simulink model "NPC_IM_YT"  (R2017b)
settings: Solver=ode45  StartTime=0.0  StopTime=5  MaxStep=1e-6  RelTol=1e-3
libraries: powerlib x35
settings Model: Creator=sibly  LastModifiedBy=alfonso
settings CodeAppCC: StateflowObjectComments=on
settings SimscapeCC: SimscapeNormalizeSystem=off

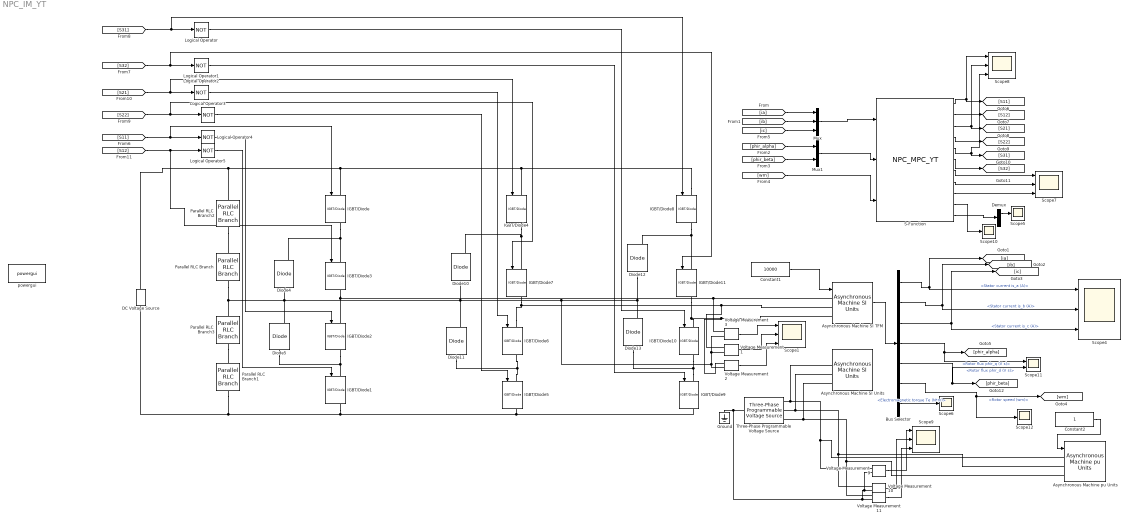
== system NPC_IM_YT ==
  Asynchronous Machine SI TFM : powerlib/Machines/Asynchronous Machine SI Units  RotorType=Squirrel-cage  PresetModel=No  MechanicalLoad=Torque Tm  ShowDetailedParameters=on  ReferenceFrame=Stationary  Units=SI  MeasurementBus=off  NominalParameters=[2035e3 3300 50]  Stator=[0.05761 0.002544]  Rotor=[0.04889 0.001881]  Cage1=[0.4155 0.002066]  Cage2=[0.4168 0.0003495]  Lm=0.04001  Mechanical=[42.14 0 5]  PolePairs=2  InitialConditions=[0 0 0 0 0 0 0 0]  SimulateSaturation=off  Saturation=[14.03593122, 27.81365428, 53.79336849, 72.68890987, 97.98006896, 148.6815601, 215.7428561, 302.9841135, 428.7778367 ; 230, 322, 414, 460, 506, 552, 598, 644, 690]  LoadFlowParameters=1492000  TsPowergui=0  TsBlock=-1  IterativeModel=Trapezoidal non iterative  IterativeDiscreteModel=Trapezoidal non iterative  Pmec=1.587e6
  Asynchronous Machine SI Units : powerlib/Machines/Asynchronous Machine SI Units  RotorType=Squirrel-cage  PresetModel=No  MechanicalLoad=Torque Tm  ShowDetailedParameters=on  ReferenceFrame=Stationary  Units=SI  MeasurementBus=off  NominalParameters=[7000 460 60]  Stator=[0.6837 0.004125]  Rotor=[0.451 0.004125]  Cage1=[0.4155 0.002066]  Cage2=[0.4168 0.0003495]  Lm=0.1486  Mechanical=[0.05 0 2]  PolePairs=2  InitialConditions=[0 0 0 0 0 0 0 0]  SimulateSaturation=off  Saturation=[14.03593122, 27.81365428, 53.79336849, 72.68890987, 97.98006896, 148.6815601, 215.7428561, 302.9841135, 428.7778367 ; 230, 322, 414, 460, 506, 552, 598, 644, 690]  LoadFlowParameters=1492000  TsPowergui=0  TsBlock=-1  IterativeModel=Trapezoidal non iterative  IterativeDiscreteModel=Trapezoidal non iterative  Pmec=1.492e+006
  Asynchronous Machine pu Units : powerlib/Machines/Asynchronous Machine pu Units  RotorType=Squirrel-cage  PresetModel=No  MechanicalLoad=Torque Tm  ShowDetailedParameters=on  ReferenceFrame=Stationary  Units=pu  MeasurementBus=off  NominalParameters=[2035e3 3300 50]  Stator=[0.0108 0.1493]  Rotor=[0.0091 0.1104]  Cage1=[0.01909 0.0397]  Cage2=[0.01909 0.0397]  Lm=2.349  Mechanical=[0.1635 0 5]  PolePairs=5  InitialConditions="[ 1,0   0,0,0   0,0,0 ]"  SimulateSaturation=off  Saturation="[0.212,0.4201,0.8125,1.0979,1.4799,2.2457,3.2586,4.5763,6.4763 ;   0.5,0.7,0.9,1,1.1,1.2 ,1.3,1.4,1.5]"  LoadFlowParameters=0  TsPowergui=0  TsBlock=-1  IterativeModel=Trapezoidal non iterative  IterativeDiscreteModel=Trapezoidal non iterative  Pmec=0
      settings: SourceProductName=Simscape Power Systems  SourceProductBaseCode=PS
  Bus Selector : BusSelector  OutputSignals=Stator measurements.Stator current is_a (A),Stator measurements.Stator current is_b (A),Stator measurements.Stator current is_c (A),Rotor measurements.Rotor flux phir_q (V s),Rotor measurements.Rotor flux phir_d (V s),Mechanical.Rotor speed (wm),Mechanical.Electromagnetic torque Te (N*m)
  Constant1 : Constant  Value=10000
  Constant2 : Constant
  DC Voltage Source : powerlib/Electrical Sources/DC Voltage Source  Amplitude=5200  Measurements=None
  Demux : Demux  Outputs=2
  Diode{4..5,10..13} (6 alike) : powerlib/Power Electronics/Diode  Ron=0.001  Lon=0  Vf=0.8  IC=0  UseSnubber=0  Rs=500  Cs=250e-9  Measurements=on
  Ground : powerlib/Elements/Ground  LConnTagsString=a
  IGBT/Diode{,1..11} (12 alike) : powerlib/Power Electronics/IGBT//Diode  Ron=1e-3  Rs=1e5  Cs=inf  Measurements=on
  Logical Operator{,1..5} (6 alike) : Logic  Operator=NOT  AllPortsSameDT=off  OutDataTypeStr=boolean
  Mux : Mux  Inputs=3
  Mux1 : Mux  Inputs=2
  Parallel RLC Branch : powerlib/Elements/Parallel RLC Branch  LConnTagsString=a  RConnTagsString=__new0  BranchType=C  Resistance=0  Inductance=0  SetiL0=off  InitialCurrent=0  Capacitance=7e-3  Setx0=off  InitialVoltage=0  Measurements=None
  Parallel RLC Branch1 : powerlib/Elements/Parallel RLC Branch  LConnTagsString=a  RConnTagsString=__new0  BranchType=C  Resistance=0  Inductance=0  SetiL0=off  InitialCurrent=0  Capacitance=7e-3  Setx0=off  InitialVoltage=0  Measurements=None
  Parallel RLC Branch2 : powerlib/Elements/Parallel RLC Branch  LConnTagsString=a  RConnTagsString=__new0  BranchType=R  Resistance=1  Inductance=0  SetiL0=off  InitialCurrent=0  Capacitance=7e-3  Setx0=off  InitialVoltage=0  Measurements=None
  Parallel RLC Branch3 : powerlib/Elements/Parallel RLC Branch  LConnTagsString=a  RConnTagsString=__new0  BranchType=R  Resistance=1  Inductance=0  SetiL0=off  InitialCurrent=0  Capacitance=7e-3  Setx0=off  InitialVoltage=0  Measurements=None
  S-Function : S-Function  FunctionName=NPC_MPC_YT  SFunctionDeploymentMode=off  EnableBusSupport=off
  Scope{1,4,7..9} (5 alike) : Scope  NumInputPorts=3
  Scope{5..6,10,12} (4 alike) : Scope
  Scope11 : Scope  NumInputPorts=2
  Three-Phase Programmable Voltage Source : powerlib/Electrical Sources/Three-Phase Programmable Voltage Source  PositiveSequence="[3300  0 50]"  VariationEntity=None  VariationType=Table of time-amplitude pairs  VariationTypeAlt=Step  VariationStep=0.5  VariationRate=10  VariationMagnitude=0.3  VariationFrequency=2  VariationTiming=[1 2]  VariationPhaseA=off  Amplitudes=[1 0.8 1.2 1.0]  TimeValues=[0 0.1 0.15 0.2]  HarmonicGeneration=off  HarmonicA=[3 0.2 -25 0]  HarmonicB=[2 0.15 35 2]  Timing="[0.05  3]"  BusType=swing  Pref=0  Qref=0  Qmin=-inf  Qmax=inf
  Voltage Measurement{1..3,9..11} (6 alike) : powerlib/Measurements/Voltage Measurement  PhasorSimulation=off  OutputType=Complex  PSBequivalent=0
  powergui : powerlib/powergui  Priority=1  SimulationMode=Continuous  SampleTime=1e-6  frequency=60  Iterations=1000  frequencyindice=50  Pbase=2.035e6  ErrMax=1e-4  UnitsV=kV  UnitsW=MW  buscounter=0  FunctionMessages=off  echomessages=off  EnableUseOfTLC=off  CurrentSourceSwitches=off  DisableSnubberDevices=off  DisableRonSwitches=off  DisableVfSwitches=off  DisplayEquations=off  SolverType=Tustin/Backward Euler (TBE)  Interpol=off  ExternalGateDelay=off  methode=off  Ts=100  x0status=blocks  SPID=on  SwTol=0  HookPort=off  RestoreLinks=warning  ResistiveCurrentMeasurement=off  Frange=[0:2:500]  Ylog=off  Xlog=on  ShowGrid=off  save=off  variable=ZData  structure=ScopeData2  ZoomFFT=off  StartTime=0.05  cycles=1  DisplayStyle=1  fundamental=50  FreqAxis=off  MaxFrequency=5000  frequencyindicesteady=1  RmsSteady=1  display=off
  wires:
  [S12] -> Logical Operator5/1, IGBT/Diode3/1
  [S11] -> Logical Operator4/1, IGBT/Diode/1
  Logical Operator4/1 -> IGBT/Diode2/1
  Logical Operator5/1 -> IGBT/Diode1/1
  [S31] -> Logical Operator/1, IGBT/Diode8/1
  [S32] -> Logical Operator1/1, IGBT/Diode11/1
  [S21] -> Logical Operator2/1, IGBT/Diode4/1
  [S22] -> Logical Operator3/1, IGBT/Diode7/1
  Logical Operator2/1 -> IGBT/Diode6/1
  Logical Operator3/1 -> IGBT/Diode5/1
  Logical Operator/1 -> IGBT/Diode10/1
  Logical Operator1/1 -> IGBT/Diode9/1
  Bus Selector/6 -> Scope12/1, [wm]  "<Rotor speed (wm)>"
  Constant1/1 -> Asynchronous Machine SI TFM/1
  [phir_beta] -> Mux1/2
  [phir_alpha] -> Mux1/1
  Mux1/1 -> S-Function/2
  [ib] -> Mux/2
  [ia] -> Mux/1
  Mux/1 -> S-Function/1
  S-Function/3 -> [S21], Scope8/2
  S-Function/2 -> [S12]
  S-Function/1 -> [S11], Scope8/1
  S-Function/5 -> [S31], Scope8/3
  S-Function/4 -> [S22]
  S-Function/6 -> [S32]
  Bus Selector/1 -> [ia], Scope4/1  "<Stator current is_a (A)>"
  Bus Selector/2 -> Scope4/2, [ib]  "<Stator current is_b (A)>"
  Bus Selector/3 -> Scope4/3, [ic]  "<Stator current is_c (A)>"
  S-Function/7 -> Scope7/1
  S-Function/8 -> Scope7/2
  S-Function/9 -> Scope7/3
  Voltage Measurement9/1 -> Scope9/1
  Voltage Measurement10/1 -> Scope9/2
  Voltage Measurement11/1 -> Scope9/3
  [wm] -> S-Function/3
  Demux/1 -> Scope5/1
  S-Function/10 -> Scope10/1
  S-Function/11 -> Demux/1
  Bus Selector/4 -> Scope11/1, [phir_alpha]  "<Rotor flux phir_q (V s)>"
  Bus Selector/5 -> Scope11/2, [phir_beta]  "<Rotor flux phir_d (V s)>"
  [ic] -> Mux/3
  Bus Selector/7 -> Scope6/1  "<Electromagnetic torque Te (N*m)>"
  Constant2/1 -> Asynchronous Machine pu Units/1
  Asynchronous Machine SI TFM/1 -> Bus Selector/1
  Voltage Measurement1/1 -> Scope1/2
  Voltage Measurement2/1 -> Scope1/3
  Voltage Measurement3/1 -> Scope1/1
  connections:
  Diode12/LConn1 -- Diode13/RConn1 -- Voltage Measurement2/LConn2 -- Voltage Measurement1/LConn2 -- Voltage Measurement3/LConn2 -- Parallel RLC Branch3/LConn1 -- Parallel RLC Branch/RConn1 -- Diode5/RConn1 -- Diode4/LConn1 -- Diode11/RConn1 -- Diode10/LConn1
  IGBT/Diode3/RConn1 -- Voltage Measurement3/LConn1 -- Asynchronous Machine SI TFM/LConn1 -- IGBT/Diode2/LConn1
  Diode5/LConn1 -- IGBT/Diode2/RConn1 -- IGBT/Diode1/LConn1
  Diode10/RConn1 -- IGBT/Diode7/LConn1 -- IGBT/Diode4/RConn1
  IGBT/Diode6/LConn1 -- Voltage Measurement1/LConn1 -- Asynchronous Machine SI TFM/LConn2 -- IGBT/Diode7/RConn1
  Diode11/LConn1 -- IGBT/Diode6/RConn1 -- IGBT/Diode5/LConn1
  Diode13/LConn1 -- IGBT/Diode10/RConn1 -- IGBT/Diode9/LConn1
  IGBT/Diode11/RConn1 -- Voltage Measurement2/LConn1 -- Asynchronous Machine SI TFM/LConn3 -- IGBT/Diode10/LConn1
  Diode12/RConn1 -- IGBT/Diode11/LConn1 -- IGBT/Diode8/RConn1
  IGBT/Diode1/RConn1 -- DC Voltage Source/LConn1 -- Parallel RLC Branch1/RConn1 -- IGBT/Diode5/RConn1 -- IGBT/Diode9/RConn1
  IGBT/Diode/RConn1 -- IGBT/Diode3/LConn1 -- Diode4/RConn1
  Three-Phase Programmable Voltage Source/LConn1 -- Voltage Measurement9/LConn2 -- Voltage Measurement10/LConn2 -- Voltage Measurement11/LConn2 -- Ground/LConn1
  IGBT/Diode8/LConn1 -- IGBT/Diode4/LConn1 -- Parallel RLC Branch2/LConn1 -- DC Voltage Source/RConn1 -- IGBT/Diode/LConn1
  Parallel RLC Branch2/RConn1 -- Parallel RLC Branch/LConn1
  Parallel RLC Branch3/RConn1 -- Parallel RLC Branch1/LConn1
  Voltage Measurement11/LConn1 -- Asynchronous Machine pu Units/LConn3 -- Asynchronous Machine SI Units/LConn3 -- Three-Phase Programmable Voltage Source/RConn3
  Voltage Measurement10/LConn1 -- Asynchronous Machine pu Units/LConn2 -- Asynchronous Machine SI Units/LConn2 -- Three-Phase Programmable Voltage Source/RConn2
  Voltage Measurement9/LConn1 -- Asynchronous Machine pu Units/LConn1 -- Asynchronous Machine SI Units/LConn1 -- Three-Phase Programmable Voltage Source/RConn1
